simulink model "motor_spacestateequation"  (R2021a)
settings: Solver=FixedStepAuto  StartTime=0.0  StopTime=10.0  FixedStep=0.001  RelTol=1e-3
libraries: pid_lib x1
settings Model: Creator=Admin  LastModifiedBy=Admin

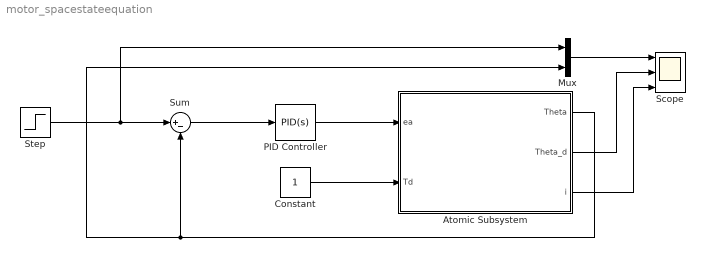
== system motor_spacestateequation ==
  Atomic Subsystem : Subsystem  TreatAsAtomicUnit=on
  Constant : Constant
  Mux : Mux  Inputs=2
  PID Controller : pid_lib/PID Controller  Controller=PID  Form=Parallel  TimeDomain=Continuous-time  UseExternalTs=off  SampleTime=-1  IntegratorMethod=Forward Euler  FilterMethod=Forward Euler  ControllerParametersSource=internal  P=5  I=0  D=2  UseFilter=on  N=100  TunerSelectOption=Transfer Function Based (PID Tuner App)  InitialConditionSource=internal  InitialConditionForIntegrator=0  InitialConditionForFilter=0  DifferentiatorICPrevScaledInput=0  ExternalReset=none  TrackingMode=off  Kt=1  LimitOutput=off  SatLimitsSource=internal  UpperSaturationLimit=inf  LowerSaturationLimit=-inf  LinearizeAsGain=on  AntiWindupMode=none  Kb=1  POutMin=[]  POutMax=[]  IOutMin=[]  IOutMax=[]  DOutMin=[]  DOutMax=[]  NOutMin=[]  NOutMax=[]  SumOutMin=[]  SumOutMax=[]  SaturationOutMin=[]  SaturationOutMax=[]  PParamMin=[]  PParamMax=[]  IParamMin=[]  IParamMax=[]  DParamMin=[]  DParamMax=[]  NParamMin=[]  NParamMax=[]  KbParamMin=[]  KbParamMax=[]  KtParamMin=[]  KtParamMax=[]  KbOutMin=[]  KbOutMax=[]  KtOutMin=[]  KtOutMax=[]  IntegratorOutMin=[]  IntegratorOutMax=[]  FilterOutMin=[]  FilterOutMax=[]  SumI1OutMin=[]  SumI1OutMax=[]  SumI2OutMin=[]  SumI2OutMax=[]  SumI3OutMin=[]  SumI3OutMax=[]  SumI4OutMin=[]  SumI4OutMax=[]  SumDOutMin=[]  SumDOutMax=[]  DifferentiatorOutMin=[]  DifferentiatorOutMax=[]  FilterDiffOutCoefMin=[]  FilterDiffOutCoefMax=[]  ReciprocalOutMin=[]  ReciprocalOutMax=[]  SumDenOutMin=[]  SumDenOutMax=[]  SumNumOutMin=[]  SumNumOutMax=[]  DivideOutMin=[]  DivideOutMax=[]  UdiffTsProdOutMin=[]  UdiffTsProdOutMax=[]  NTsProdOutMin=[]  NTsProdOutMax=[]  UintegralTsProdOutMin=[]  UintegralTsProdOutMax=[]  UngainTsProdOutMin=[]  UngainTsProdOutMax=[]  IntegratorContinuousStateAttributes=''  IntegratorStateMustResolveToSignalObject=off  IntegratorRTWStateStorageClass=Auto  FilterContinuousStateAttributes=''  FilterStateMustResolveToSignalObject=off  FilterRTWStateStorageClass=Auto  ParallelPVariant=InternalParameters  IdealPVariant=Disabled  IVariant=InternalParameters  DVariant=InternalParameters  IntegratorVariant=Continuous  SatVariant=Disabled  AWVariant=Passthrough  PCopyVariant=Disabled  TRVariant=Disabled  FdbkBlocksVariant=Forward  IdealPFdbkVariant=Disabled  SatFdbkVariant=Disabled  DerivativeFilterVariant=ContFilter  NVariant=InternalParameters  NCopyVariant=Disabled  FilterICVariant=InternalICsFilter  IntegratorICVariant=InternalICs  ExternalResetVariant=Disabled  TRSumVariant=Passthrough  SumFdbkVariant=Disabled  SumVariant=Sum_PID  TsampFilterVariant=InternalTs  TsampNgainVariant=Passthrough  TsampIntegralVariant=Passthrough  ExternalSaturationOutDataTypeStr=Inherit: Same as second input
  Scope : Scope  NumInputPorts=3
  Step : Step  Time=0  After=200  SampleTime=0
  Sum : Sum  Inputs=|+-
  wires:
  Constant/1 -> Atomic Subsystem/2(Td)
  Atomic Subsystem/1(Theta) -> Mux/2, Sum/2
  Step/1 -> Mux/1, Sum/1
  Sum/1 -> PID Controller/1
  PID Controller/1 -> Atomic Subsystem/1(ea)
  Atomic Subsystem/2(Theta_d) -> Scope/2
  Atomic Subsystem/3(i) -> Scope/3
  Mux/1 -> Scope/1

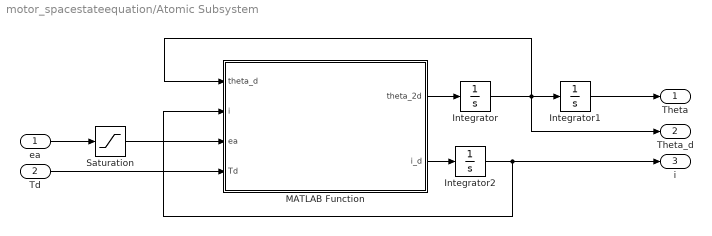
== system motor_spacestateequation/Atomic Subsystem ==
  ea : Inport
  Td : Inport  Port=2
  Integrator : Integrator
  Integrator1 : Integrator
  Integrator2 : Integrator
  MATLAB Function : MATLAB Function  TreatAsAtomicUnit=on
  Saturation : Saturate
  Theta : Outport
  Theta_d : Outport  Port=2
  i : Outport  Port=3
  wires:
  Saturation/1 -> MATLAB Function/3(ea)
  MATLAB Function/1(theta_2d) -> Integrator/1
  Integrator/1 -> MATLAB Function/1(theta_d), Integrator1/1, Theta_d/1
  MATLAB Function/2(i_d) -> Integrator2/1
  Td/1 -> MATLAB Function/4(Td)
  Integrator2/1 -> MATLAB Function/2(i), i/1
  ea/1 -> Saturation/1
  Integrator1/1 -> Theta/1

== matlab function motor_spacestateequation/Atomic Subsystem/MATLAB Function ==
  data: theta_d input; theta_2d output; i input; ea input; Td input; i_d output
function [theta_2d,i_d] = DC_Motor(theta_d,i,ea,Td)
%% Declare the parameters
Ra=2;
La=0.5;
Jm=0.02;
Dm=0.002953;
Kt=1.28;
Kb=0.0015;
%% System differential equations:
i_d=1/La*ea-Kb*La-theta_d-Ra/La*i;
theta_2d=Kt/Jm*i-Dm/Jm*theta_d-Td;
